simulink model "PID_mode"  (R2020a)
settings: Solver=FixedStepAuto  StartTime=0.0  StopTime=100  RelTol=1e-3
undefined symbols (not defined in the file or in its folder): Kd, Ki, Kp
settings Model: Creator=sun  LastModifiedBy=sun
settings SolverCC: ZeroCrossAlgorithm=Adaptive
settings DebuggingCC: IgnoredZcDiagnostic=none

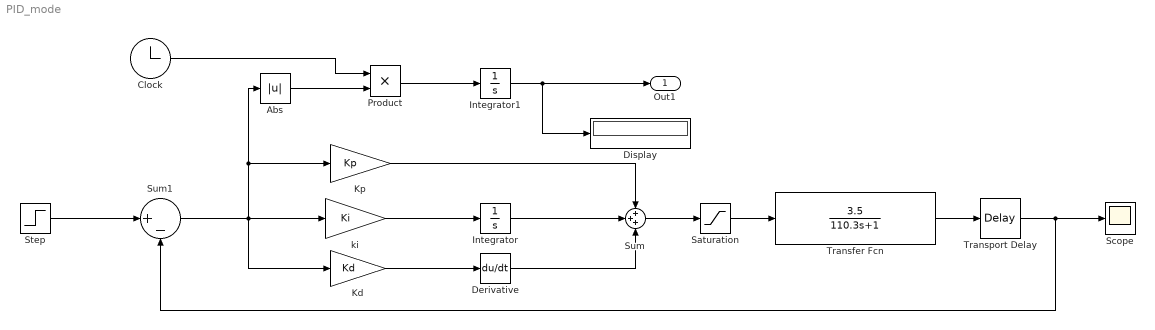
== system PID_mode ==
  Abs : Abs
  Clock : Clock
  Derivative : Derivative
  Display : Display
  Integrator : Integrator
  Integrator1 : Integrator
  Kd : Gain  Gain=Kd
  Kp : Gain  Gain=Kp
  Product : Product
  Saturation : Saturate  UpperLimit=5  LowerLimit=-5
  Scope : Scope
  Step : Step  Time=0  SampleTime=0
  Sum : Sum  Inputs=+++
  Sum1 : Sum  Inputs=|+-
  Transfer Fcn : TransferFcn  Numerator=[3.5]  Denominator=[110.3 1]
  Transport Delay : TransportDelay  DelayTime=2  BufferSize=2048
  ki : Gain  Gain=Ki
  Out1 : Outport
  wires:
  Clock/1 -> Product/1
  Abs/1 -> Product/2
  Product/1 -> Integrator1/1
  Integrator1/1 -> Display/1, Out1/1
  Step/1 -> Sum1/1
  Derivative/1 -> Sum/3
  Integrator/1 -> Sum/2
  Kp/1 -> Sum/1
  Sum/1 -> Saturation/1
  Kd/1 -> Derivative/1
  ki/1 -> Integrator/1
  Sum1/1 -> Kd/1, ki/1, Abs/1, Kp/1
  Transfer Fcn/1 -> Transport Delay/1
  Saturation/1 -> Transfer Fcn/1
  Transport Delay/1 -> Scope/1, Sum1/2
